simulink model "leader"  (R2020b)
settings: Solver=VariableStepAuto  StartTime=0.0  StopTime=time  MaxStep=1e-3  RelTol=1e-3
values from neighbouring files (symbols this model uses):
  A_plant = [0 1; 880.87 0]    [alternative_model.m]    (also in alternative_model_script.m; observer_convergence.m; p1.m; stable_template.m)
  B_plant = [0; -9.9453]    [alternative_model.m]    (also in alternative_model_script.m; observer_convergence.m; p1.m; stable_template.m)
  C_plant = [708.27 0]    [alternative_model.m]    (also in alternative_model_script.m; observer_convergence.m; p1.m; stable_template.m)
  K_plant = acker(A_plant, B_plant, poles)    [alternative_model.m]    (also in alternative_model_script.m; p1.m; stable_template.m; template.m)
  x0_leader = [1e-3 1e-3]    [alternative_model.m]    (also in alternative_model_script.m; p1.m = [100 0]; stable_template.m = [.1 0]; template.m = [0 0])
libraries: cstblocks x1
settings Model: Creator=salvo  LastModifiedBy=salvo

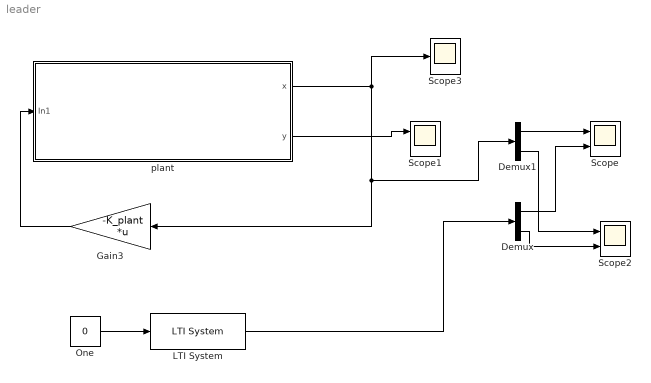
== system leader ==
  Demux : Demux  Outputs=2
  Demux1 : Demux  Outputs=2
  Gain3 : Gain  Gain=-K_plant  Multiplication=Matrix(K*u)
  LTI System : cstblocks/LTI System  sys=sys  IC=x0_leader
  One : Constant  Value=0  OutDataTypeStr=Inherit: Inherit via back propagation
  Scope : Scope  NumInputPorts=2
  Scope1 : Scope  NumInputPorts=2
  Scope2 : Scope  NumInputPorts=2
  Scope3 : Scope
  plant : Subsystem
  wires:
  plant/1(x) -> Scope3/1, Demux1/1, Gain3/1
  plant/2(y) -> Scope1/1
  One/1 -> LTI System/1
  Demux1/1 -> Scope/1
  LTI System/1 -> Demux/1
  Demux/1 -> Scope/2
  Demux1/2 -> Scope2/1
  Demux/2 -> Scope2/2
  Gain3/1 -> plant/1(In1)

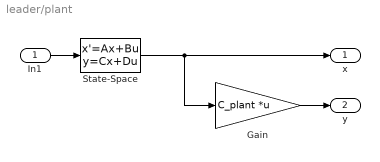
== system leader/plant ==
  In1 : Inport
  Gain : Gain  Gain=C_plant  Multiplication=Matrix(K*u)
  State-Space : StateSpace  A=A_plant  B=B_plant  C=eye(2)  D=[0; 0]  InitialCondition=x0_leader
  x : Outport  PortDimensions=[2,1]
  y : Outport  Port=2  PortDimensions=1
  wires:
  In1/1 -> State-Space/1
  Gain/1 -> y/1
  State-Space/1 -> x/1, Gain/1
